simulink model "counter"  (R2017a)
settings: Solver=FixedStepDiscrete  StartTime=0.0  StopTime=10.0  RelTol=1e-3
settings Model: Creator=rober  LastModifiedBy=rober

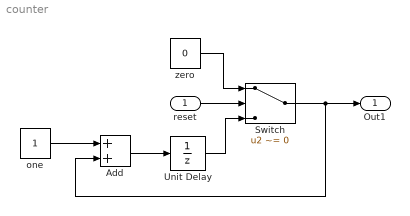
== system counter ==
  reset : Inport  OutDataTypeStr=boolean
  Add : Sum  OutDataTypeStr=uint32
  Switch : Switch  Criteria=u2 ~= 0
  Unit Delay : UnitDelay  SampleTime=-1
  one : Constant  OutDataTypeStr=uint32
  zero : Constant  Value=0  OutDataTypeStr=uint32
  Out1 : Outport
  wires:
  Add/1 -> Unit Delay/1
  one/1 -> Add/1
  Switch/1 -> Add/2, Out1/1
  zero/1 -> Switch/1
  Unit Delay/1 -> Switch/3
  reset/1 -> Switch/2
